simulink subsystem "BatteryTableBased"  (R2024b)
settings: Solver=VariableStepAuto  StartTime=0.0  StopTime=10.0  RelTol=1e-3
undefined symbols (not defined in the file or in its folder): battery
libraries: fl_lib x17, nesl_utility x9, batteryecm_lib x1, simulink x1
Description:
  | Battery Table-Based (Thermal)
  | 
  | ⚡ Main Features:
  | - Positive & negative relays for HV bus connection
  | - Electrical behavior from lookup tables (SOC–OCV, resistance vs SOC/Temp)
  | - Thermal port for coolant/heater coupling
  | - Voltage & current sensors for measurement
  | - Status bus bundles key signals
  | 
  | 📤 Outputs: Voltage, Current, SOC, Cell Voltage, Temperature
  | 
  | 📌 Use Case: High-fidelity drive cycle and thermal management studies
settings Model: Creator=isaacito  LastModifiedBy=jjha
settings OptimizationCC: ReuseModelBlockBuffer=off
settings RTWCC: GPUComputeCapability=3.5

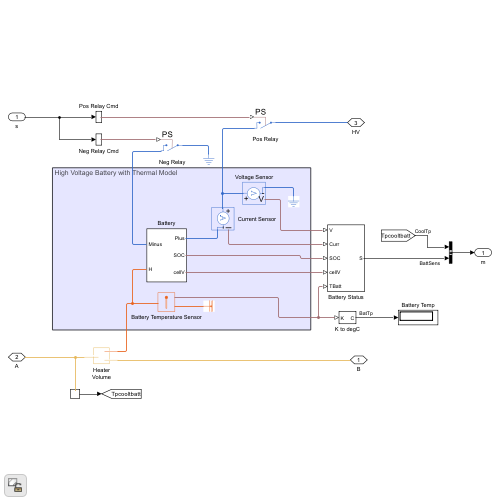
[thumbnail: Simulink's stored preview of the top-level diagram]
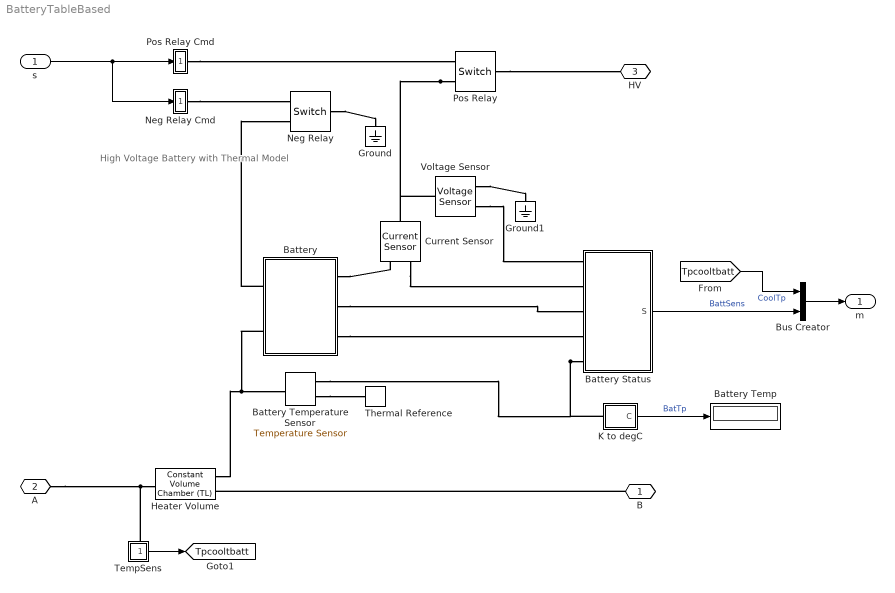
== system BatteryTableBased ==
  note: High Voltage Battery with Thermal Model
  s : Inport
  Battery : Subsystem
  Battery Status : Subsystem
  Battery Temp : Display
  Battery Temperature Sensor : fl_lib/Thermal/Thermal Sensors/Temperature Sensor  temperature_measure=foundation.enum.MeasurementReference.difference
  Bus Creator : BusCreator  Inputs=2
  Current Sensor : fl_lib/Electrical/Electrical Sensors/Current Sensor
  Ground : fl_lib/Electrical/Electrical Elements/Electrical Reference
  Ground1 : fl_lib/Electrical/Electrical Elements/Electrical Reference
  Heater Volume : fl_lib/Thermal Liquid/Elements/Constant Volume Chamber (TL)  volume=0.003 m^3  num_ports=foundation.enum.num_ports.two  area_A=pi * battery.coolant_pipe_D^2 / 4 m^2  area_B=pi * battery.coolant_pipe_D^2 / 4 m^2  area_C=0.01 m^2  area_D=0.01 m^2  p_I_specify=on  p_I_priority=High  p_I=vehicleThermal.coolant_p_init MPa  p_I_nominal_specify=off  p_I_nominal_value=1  p_I_nominal_unit=MPa  T_I_specify=on  T_I_priority=Low  T_I=vehicleThermal.coolant_T_init K  T_I_nominal_specify=off  T_I_nominal_value=1  T_I_nominal_unit=K  u_I_specify=off  u_I_priority=None  u_I=83.90600000000001 kJ/kg  u_I_nominal_specify=off  u_I_nominal_value=1  u_I_nominal_unit=kJ/kg  rho_I_specify=off  rho_I_priority=None  rho_I=998.21 kg/m^3  rho_I_nominal_specify=off  rho_I_nominal_value=1  rho_I_nominal_unit=kg/m^3
      settings: InternalSimscapePortConfiguration="{\"Bottom\":[],\"Left\":[{\"id\":\"A\",\"label\":\"A\",\"type\":\"foundation.thermal_liquid.thermal_liquid\"},{\"id\":\"H\",\"label\":\"H\",\"type\":\"foundation.thermal.thermal\"}],\"Right\":[{\"id\":\"B\",\"label\":\"B\",\"type\":\"foundation.thermal_liquid.thermal_liquid\"}],\"Top\":[]}"
  K to degC : Subsystem
  Neg Relay : fl_lib/Electrical/Electrical Elements/Switch  R_closed=0.001 Ohm  G_open=1e-8 1/Ohm  Threshold=0.5  i_specify=off  i_priority=None  i=0 A  i_nominal_specify=off  i_nominal_value=1  i_nominal_unit=A  v_specify=off  v_priority=None  v=0 V  v_nominal_specify=off  v_nominal_value=1  v_nominal_unit=V
  Neg Relay Cmd : Subsystem
  Pos Relay : fl_lib/Electrical/Electrical Elements/Switch  R_closed=0.001 Ohm  G_open=1e-8 1/Ohm  Threshold=0.5  i_specify=off  i_priority=None  i=0 A  i_nominal_specify=off  i_nominal_value=1  i_nominal_unit=A  v_specify=off  v_priority=None  v=0 V  v_nominal_specify=off  v_nominal_value=1  v_nominal_unit=V
  Pos Relay Cmd : Subsystem
  TempSens : Subsystem
      settings: PortSchema="{\"entries\":[{\"content\":{\"sides\":[{\"content\":{\"connectorIds\":[]},\"type\":\"ConnectorPlacement.EquallySpacedRectSide\",\"uuid\":\"72721b76-a3c2-4898-b03f-ac2748712f42\"},{\"content\":{\"connectorIds\":[\"Out1\"],\"side\":\"RIGHT\"},\"type\":\"ConnectorPlacement.EquallySpacedRectSide\",\"uuid\":\"bc8f9114-f4be-4e78-a030-a27ecd6c9d73\"},{\"content\":{\"connectorIds\":[\"LConn1\"],\"side\":\"TOP\"},\"type\":\"ConnectorPlacement.EquallySpacedRectSide\",\"uuid\":\"2039c7b0-1e2d-4162-8de8-f9f63ba2bad7\"}]},\"type\":\"ConnectorPlacement.EquallySpacedConnector\",\"uuid\":\"7ff72b7c-043d-4221-97f0-b3933d031f4d\"}],\"packageUris\":[\"http://schema.mathworks.com/mf0/Connector/R2020b\"],\"version\":\"1.0\"}"
  Thermal Reference : fl_lib/Thermal/Thermal Elements/Thermal Reference
  Voltage Sensor : fl_lib/Electrical/Electrical Sensors/Voltage Sensor
  B : PMIOPort  Side=Left
  A : PMIOPort  Port=2  Side=Right
  HV : PMIOPort  Port=3  Side=Right
  m : Outport
  tag scope: Tpcooltbatt=global
  wires:
  s/1 -> Neg Relay Cmd/1("  "), Pos Relay Cmd/1("  ")
  TempSens/1("  ") -> [Tpcooltbatt]
  [Tpcooltbatt] -> Bus Creator/1  "CoolTp"
  Bus Creator/1 -> m/1
  Battery Status/1(S) -> Bus Creator/2  "BattSens"
  K to degC/1(C) -> Battery Temp/1  "BatTp"
  connections:
  Pos Relay/RConn2 -- Current Sensor/LConn1 -- Voltage Sensor/LConn1
  Heater Volume/LConn2 -- Battery Temperature Sensor/LConn1 -- Battery/RConn2
  Battery Status/LConn5 -- K to degC/LConn1 -- Battery Temperature Sensor/RConn2
  TempSens/LConn1 -- A/RConn1 -- Heater Volume/RConn1
  Battery/RConn1 -- Neg Relay/RConn2
  Voltage Sensor/RConn1 -- Battery Status/LConn1
  Battery Temperature Sensor/RConn1 -- Thermal Reference/LConn1
  Battery/LConn2 -- Battery Status/LConn3
  Pos Relay Cmd/RConn1 -- Pos Relay/RConn1
  Neg Relay Cmd/RConn1 -- Neg Relay/RConn1
  Neg Relay/LConn1 -- Ground/LConn1
  B/RConn1 -- Heater Volume/LConn1
  Battery/LConn3 -- Battery Status/LConn4
  Pos Relay/LConn1 -- HV/RConn1
  Battery/LConn1 -- Current Sensor/RConn2
  Current Sensor/RConn1 -- Battery Status/LConn2
  Voltage Sensor/RConn2 -- Ground1/LConn1

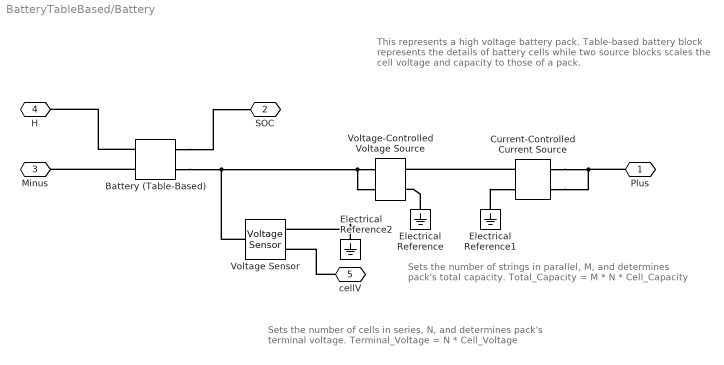
== system BatteryTableBased/Battery ==
  note: This represents a high voltage battery pack.
      | Table-based battery block represents the details of
      | battery cells while two source blocks scales
      | the cell voltage and capacity to those of a pack.
  note: Sets the number of strings in parallel, M,
      | and determines pack's total capacity.
      | Total_Capacity = M * N * Cell_Capacity
  note: Sets the number of cells in series, N,
      | and determines pack's terminal voltage.
      | Terminal_Voltage = N * Cell_Voltage
  Battery (Table-Based) : batteryecm_lib/Battery (Table-Based)  SOC_vec=battery.SOC_vec  T_dependence=simscape.enum.tablebattery.temperature_dependence.yes  prm_dir=simscape.enum.tablebattery.prm_dir.noCurrentDirectionality  T_vec=battery.T_vec K  V0_mat=battery.V0_mat V  V0_vec=[3.5057, 3.566, 3.6337, 3.7127, 3.9259, 4.0777, 4.1928] V  V_range=[0, inf] V  R0_mat=battery.R0_mat Ohm  R0_vec=[.0085, .0085, .0087, .0082, .0083, .0085, .0085] Ohm  R0_dis_mat=[.0117, .0085, .009; .011, .0085, .009; .0114, .0087, .0092; .0107, .0082, .0088; .0107, .0083, .0091; .0113, .0085, .0089; .0116, .0085, .0089] Ohm  R0_dis_vec=[.0085, .0085, .0087, .0082, .0083, .0085, .0085] Ohm  R0_ch_mat=[.0117, .0085, .009; .011, .0085, .009; .0114, .0087, .0092; .0107, .0082, .0088; .0107, .0083, .0091; .0113, .0085, .0089; .0116, .0085, .0089] Ohm  R0_ch_vec=[.0085, .0085, .0087, .0082, .0083, .0085, .0085] Ohm  AH=battery.AH A*hr  prm_leak=simscape.enum.tablebattery.prm_leak.disabled  Rleak_vec=[8000, 7000, 6000] Ohm  Rleak=7e3 Ohm  extrapolation_option=simscape.enum.extrapolation.nearest  SOC_port=simscape.enum.tablebattery.enable.yes  prm_dyn=simscape.enum.tablebattery.prm_dyn.off  R1_mat=[.0109, .0029, .0013; .0069, .0024, .0012; .0047, .0026, .0013; .0034, .0016, .001; .0033, .0023, .0014; .0033, .0018, .0011; .0028, .0017, .0011] Ohm  R1_vec=[.0029, .0024, .0026, .0016, .0023, .0018, .0017] Ohm  tau1_mat=[20, 36, 39; 31, 45, 39; 109, 105, 61; 36, 29, 26; 59, 77, 67; 40, 33, 29; 25, 39, 33] s  tau1_vec=[36, 45, 105, 29, 77, 33, 39] s  R2_mat=[.0109, .0029, .0013; .0069, .0024, .0012; .0047, .0026, .0013; .0034, .0016, .001; .0033, .0023, .0014; .0033, .0018, .0011; .0028, .0017, .0011] Ohm  R2_vec=[.0029, .0024, .0026, .0016, .0023, .0018, .0017] Ohm  tau2_mat=[20, 36, 39; 31, 45, 39; 109, 105, 61; 36, 29, 26; 59, 77, 67; 40, 33, 29; 25, 39, 33] s  tau2_vec=[36, 45, 105, 29, 77, 33, 39] s  R3_mat=[.0109, .0029, .0013; .0069, .0024, .0012; .0047, .0026, .0013; .0034, .0016, .001; .0033, .0023, .0014; .0033, .0018, .0011; .0028, .0017, .0011] Ohm  R3_vec=[.0029, .0024, .0026, .0016, .0023, .0018, .0017] Ohm  tau3_mat=[20, 36, 39; 31, 45, 39; 109, 105, 61; 36, 29, 26; 59, 77, 67; 40, 33, 29; 25, 39, 33] s  tau3_vec=[36, 45, 105, 29, 77, 33, 39] s  R4_mat=[.0109, .0029, .0013; .0069, .0024, .0012; .0047, .0026, .0013; .0034, .0016, .001; .0033, .0023, .0014; .0033, .0018, .0011; .0028, .0017, .0011] Ohm  R4_vec=[.0029, .0024, .0026, .0016, .0023, .0018, .0017] Ohm  tau4_mat=[20, 36, 39; 31, 45, 39; 109, 105, 61; 36, 29, 26; 59, 77, 67; 40, 33, 29; 25, 39, 33] s  tau4_vec=[36, 45, 105, 29, 77, 33, 39] s  R5_mat=[.0109, .0029, .0013; .0069, .0024, .0012; .0047, .0026, .0013; .0034, .0016, .001; .0033, .0023, .0014; .0033, .0018, .0011; .0028, .0017, .0011] Ohm  R5_vec=[.0029, .0024, .0026, .0016, .0023, .0018, .0017] Ohm  tau5_mat=[20, 36, 39; 31, 45, 39; 109, 105, 61; 36, 29, 26; 59, 77, 67; 40, 33, 29; 25, 39, 33] s  tau5_vec=[36, 45, 105, 29, 77, 33, 39] s  prm_fade=simscape.enum.tablebattery.prm_fade.disabled  N0=100  dV0=0  dR0=0  dAH=0  dRleak=0  dR1=0  dR2=0  dR3=0  dR4=0  dR5=0  N0vec=[100, 200, 300]  Tfadevec=[298.15, 323.15] K  dV0vec=[0, 0, 0]  dR0vec=[0, 0, 0]  dAHvec=[0, 0, 0]  dRleakvec=[0, 0, 0]  dR1vec=[0, 0, 0]  dR2vec=[0, 0, 0]  dR3vec=[0, 0, 0]  dR4vec=[0, 0, 0]  dR5vec=[0, 0, 0]  dV0mat=[0, 0; 0, 0; 0, 0]  dR0mat=[0, 0; 0, 0; 0, 0]  dAHmat=[0, 0; 0, 0; 0, 0]  dRleakmat=[0, 0; 0, 0; 0, 0]  dR1mat=[0, 0; 0, 0; 0, 0]  dR2mat=[0, 0; 0, 0; 0, 0]  dR3mat=[0, 0; 0, 0; 0, 0]  dR4mat=[0, 0; 0, 0; 0, 0]  dR5mat=[0, 0; 0, 0; 0, 0]  prm_age_modeling=simscape.enum.tablebattery.prm_age_modeling.equation  storage_dt_age_vec=[0] d  storage_T_age_vec=[273] K  prm_age_OCV=simscape.enum.tablebattery.prm_age_OCV.OCV  OCV_age=0.9  SOC_age=0.6  prm_age_resistance=simscape.enum.tablebattery.prm_age.disabled  OCV_scaling_age_resistance=2.2134e6  OCV_offset_age_resistance=1.632e6  temp_exp_age_resistance=0.515833569 V  t_exp_age_resistance=0.75  T_age_vec_resistance=[273.15, 298.15, 323.15] K  dt_age_vec_resistance=[90, 180, 270, 360] d  dR0_age_vec=[0, 0, 0]  t_meas_dR0_age=100 d  dR0_age_mat=[0, 0, 0; 0, 0, 0; 0, 0, 0; 0, 0, 0]  prm_age_capacity=simscape.enum.tablebattery.prm_age.disabled  OCV_scaling_age_capacity=1.5097e07  OCV_offset_age_capacity=8.3625e06  temp_exp_age_capacity=0.6011 V  t_exp_age_capacity=0.75  T_age_vec_capacity=[273.15, 298.15, 323.15] K  dt_age_vec_capacity=[90, 180, 270, 360] d  dAH_age_vec=[0, 0, 0]  t_meas_dAH_age=100 d  dAH_age_mat=[0, 0, 0; 0, 0, 0; 0, 0, 0; 0, 0, 0]  thermal_port=simscape.enum.thermaleffects.model  temperature=298.15 K  thermal_mass=battery.Ns J/K  i_specify=off  i_priority=None  i=0 A  i_nominal_specify=off  i_nominal_value=1  i_nominal_unit=A  v_specify=off  v_priority=None  v=0 V  v_nominal_specify=off  v_nominal_value=1  v_nominal_unit=V  stateOfCharge_specify=on  stateOfCharge_priority=High  stateOfCharge=battery.initialPackSOC  stateOfCharge_nominal_specify=off  stateOfCharge_nominal_value=1  stateOfCharge_nominal_unit=1  num_cycles_specify=off  num_cycles_priority=High  num_cycles=0  num_cycles_nominal_specify=off  num_cycles_nominal_value=1  num_cycles_nominal_unit=1  cell_temperature_specify=on  cell_temperature_priority=Low  cell_temperature=vehicleThermal.ambient K  cell_temperature_nominal_specify=off  cell_temperature_nominal_value=1  cell_temperature_nominal_unit=K
  Current-Controlled Current Source : fl_lib/Electrical/Electrical Sources/Current-Controlled Current Source  K=battery.Np*-1  i1_specify=off  i1_priority=None  i1=0 A  i1_nominal_specify=off  i1_nominal_value=1  i1_nominal_unit=A  i2_specify=off  i2_priority=None  i2=0 A  i2_nominal_specify=off  i2_nominal_value=1  i2_nominal_unit=A
      settings: InternalSimscapePortConfiguration="{\"Bottom\":[],\"Left\":[{\"id\":\"p1\",\"label\":\"+\",\"type\":\"foundation.electrical.electrical\"},{\"id\":\"head\",\"label\":\"\",\"type\":\"foundation.electrical.electrical\"}],\"Right\":[{\"id\":\"n1\",\"label\":\"-\",\"type\":\"foundation.electrical.electrical\"},{\"id\":\"tail\",\"label\":\"\",\"type\":\"foundation.electrical.electrical\"}],\"Top\":[]}"
  Electrical Reference : fl_lib/Electrical/Electrical Elements/Electrical Reference
  Electrical Reference1 : fl_lib/Electrical/Electrical Elements/Electrical Reference
  Electrical Reference2 : fl_lib/Electrical/Electrical Elements/Electrical Reference
  Voltage Sensor : fl_lib/Electrical/Electrical Sensors/Voltage Sensor
  Voltage-Controlled Voltage Source : fl_lib/Electrical/Electrical Sources/Voltage-Controlled Voltage Source  K=battery.Ns*-1  v1_specify=off  v1_priority=None  v1=0 V  v1_nominal_specify=off  v1_nominal_value=1  v1_nominal_unit=V  v2_specify=off  v2_priority=None  v2=0 V  v2_nominal_specify=off  v2_nominal_value=1  v2_nominal_unit=V
      settings: InternalSimscapePortConfiguration="{\"Bottom\":[],\"Left\":[{\"id\":\"p1\",\"label\":\"+\",\"type\":\"foundation.electrical.electrical\"},{\"id\":\"p2\",\"label\":\"+\",\"type\":\"foundation.electrical.electrical\"}],\"Right\":[{\"id\":\"n1\",\"label\":\"-\",\"type\":\"foundation.electrical.electrical\"},{\"id\":\"n2\",\"label\":\"-\",\"type\":\"foundation.electrical.electrical\"}],\"Top\":[]}"
  Plus : PMIOPort  Side=Left
  SOC : PMIOPort  Port=2  Side=Left
  Minus : PMIOPort  Port=3  Side=Right
  H : PMIOPort  Port=4  Side=Right
  cellV : PMIOPort  Port=5  Side=Left
  connections:
  Electrical Reference1/LConn1 -- Current-Controlled Current Source/LConn2
  Electrical Reference/LConn1 -- Voltage-Controlled Voltage Source/LConn1
  Voltage Sensor/LConn1 -- Battery (Table-Based)/LConn1 -- Voltage-Controlled Voltage Source/RConn1 -- Voltage-Controlled Voltage Source/RConn2
  Current-Controlled Current Source/LConn1 -- Voltage-Controlled Voltage Source/LConn2
  Plus/RConn1 -- Current-Controlled Current Source/RConn1 -- Current-Controlled Current Source/RConn2
  Battery (Table-Based)/RConn1 -- Minus/RConn1
  Battery (Table-Based)/LConn2 -- SOC/RConn1
  Battery (Table-Based)/RConn2 -- H/RConn1
  Electrical Reference2/LConn1 -- Voltage Sensor/RConn2
  cellV/RConn1 -- Voltage Sensor/RConn1

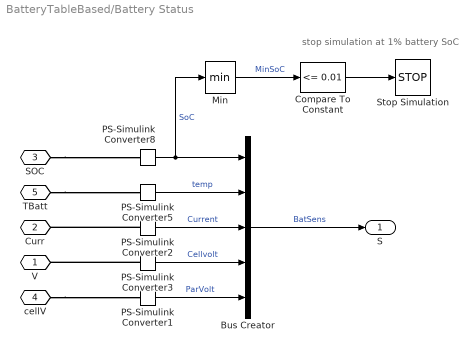
== system BatteryTableBased/Battery Status ==
  note: stop simulation at 1% battery SoC
  Bus Creator : BusCreator  Inputs=5
  Compare To Constant : simulink/Logic and Bit Operations/Compare To Constant  relop=<=  const=0.01  OutDataTypeStr=boolean
  Min : MinMax
  PS-Simulink Converter1 : nesl_utility/PS-Simulink Converter  PhysicalDomain=network_engine_domain  SubClassName=ps_output  LeftPortType=input  RightPortType=output  PseudoPeriodic=off  Frequencies=[]  VectorFormat=1-D array  Unit=V  AffineConversion=off
  PS-Simulink Converter2 : nesl_utility/PS-Simulink Converter  PhysicalDomain=network_engine_domain  SubClassName=ps_output  LeftPortType=input  RightPortType=output  PseudoPeriodic=off  Frequencies=[]  VectorFormat=1-D array  Unit=A  AffineConversion=off
  PS-Simulink Converter3 : nesl_utility/PS-Simulink Converter  PhysicalDomain=network_engine_domain  SubClassName=ps_output  LeftPortType=input  RightPortType=output  PseudoPeriodic=off  Frequencies=[]  VectorFormat=1-D array  Unit=V  AffineConversion=off
  PS-Simulink Converter5 : nesl_utility/PS-Simulink Converter  PhysicalDomain=network_engine_domain  SubClassName=ps_output  LeftPortType=input  RightPortType=output  PseudoPeriodic=off  Frequencies=[]  VectorFormat=inherit  Unit=K  AffineConversion=on
  PS-Simulink Converter8 : nesl_utility/PS-Simulink Converter  PhysicalDomain=network_engine_domain  SubClassName=ps_output  LeftPortType=input  RightPortType=output  PseudoPeriodic=off  Frequencies=[]  VectorFormat=1-D array  Unit=1  AffineConversion=off
  Stop Simulation : Stop
  V : PMIOPort  Side=Left
  Curr : PMIOPort  Port=2  Side=Left
  SOC : PMIOPort  Port=3  Side=Left
  cellV : PMIOPort  Port=4  Side=Left
  TBatt : PMIOPort  Port=5  Side=Left
  S : Outport
  wires:
  PS-Simulink Converter5/1 -> Bus Creator/2  "temp"
  PS-Simulink Converter2/1 -> Bus Creator/3  "Current"
  PS-Simulink Converter3/1 -> Bus Creator/4  "Cellvolt"
  Compare To Constant/1 -> Stop Simulation/1
  Min/1 -> Compare To Constant/1  "MinSoC"
  PS-Simulink Converter8/1 -> Min/1, Bus Creator/1  "SoC"
  PS-Simulink Converter1/1 -> Bus Creator/5  "ParVolt"
  Bus Creator/1 -> S/1  "BatSens"
  connections:
  TBatt/RConn1 -- PS-Simulink Converter5/LConn1
  SOC/RConn1 -- PS-Simulink Converter8/LConn1
  PS-Simulink Converter2/LConn1 -- Curr/RConn1
  PS-Simulink Converter3/LConn1 -- V/RConn1
  cellV/RConn1 -- PS-Simulink Converter1/LConn1

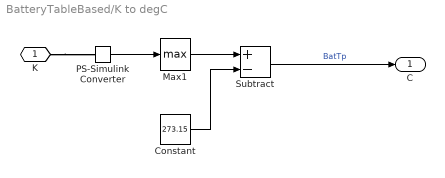
== system BatteryTableBased/K to degC ==
  Constant : Constant  Value=273.15
  Max1 : MinMax  Function=max
  PS-Simulink Converter : nesl_utility/PS-Simulink Converter  PhysicalDomain=network_engine_domain  SubClassName=ps_output  LeftPortType=input  RightPortType=output  PseudoPeriodic=off  Frequencies=[]  VectorFormat=inherit  Unit=K  AffineConversion=off
  Subtract : Sum  Inputs=+-
  K : PMIOPort  Side=Left
  C : Outport
  wires:
  PS-Simulink Converter/1 -> Max1/1
  Max1/1 -> Subtract/1
  Subtract/1 -> C/1  "BatTp"
  Constant/1 -> Subtract/2
  connections:
  K/RConn1 -- PS-Simulink Converter/LConn1

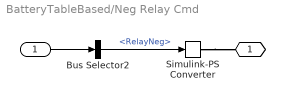
== system BatteryTableBased/Neg Relay Cmd ==
  "  " : Inport
  Bus Selector2 : BusSelector  OutputSignals=RelayNeg
  Simulink-PS Converter : nesl_utility/Simulink-PS Converter  PhysicalDomain=network_engine_domain  SubClassName=ps_input  LeftPortType=input  RightPortType=output  PseudoPeriodic=off  Frequencies=[]  NoiseDistribution=none  NoiseParameters=[]  Unit=1  AffineConversion=off  FilteringAndDerivatives=provide  SimscapeFilterOrder=1  InputFilterTimeConstant=0.001  UdotUserProvided=0
  " " : PMIOPort  Side=Right
  wires:
  "  "/1 -> Bus Selector2/1
  Bus Selector2/1 -> Simulink-PS Converter/1  "<RelayNeg>"
  connections:
  Simulink-PS Converter/RConn1 -- " "/RConn1

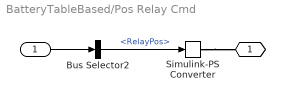
== system BatteryTableBased/Pos Relay Cmd ==
  "  " : Inport
  Bus Selector2 : BusSelector  OutputSignals=RelayPos
  Simulink-PS Converter : nesl_utility/Simulink-PS Converter  PhysicalDomain=network_engine_domain  SubClassName=ps_input  LeftPortType=input  RightPortType=output  PseudoPeriodic=off  Frequencies=[]  NoiseDistribution=none  NoiseParameters=[]  Unit=1  AffineConversion=off  FilteringAndDerivatives=provide  SimscapeFilterOrder=1  InputFilterTimeConstant=0.001  UdotUserProvided=0
  " " : PMIOPort  Side=Right
  wires:
  Bus Selector2/1 -> Simulink-PS Converter/1  "<RelayPos>"
  "  "/1 -> Bus Selector2/1
  connections:
  Simulink-PS Converter/RConn1 -- " "/RConn1

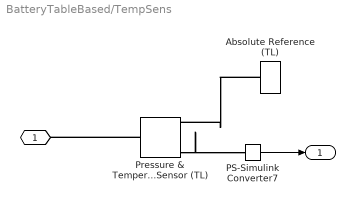
== system BatteryTableBased/TempSens ==
  Absolute Reference (TL) : fl_lib/Thermal Liquid/Elements/Absolute Reference (TL)
  PS-Simulink Converter7 : nesl_utility/PS-Simulink Converter  PhysicalDomain=network_engine_domain  SubClassName=ps_output  LeftPortType=input  RightPortType=output  PseudoPeriodic=off  Frequencies=[]  VectorFormat=inherit  Unit=inherit  AffineConversion=off
  Pressure & Temperature Sensor (TL) : fl_lib/Thermal Liquid/Sensors/Pressure & Temperature Sensor (TL)  reference=foundation.enum.MeasurementReference.difference  pressure=true  pressure_spec=foundation.enum.PressureMeasementSpec.Absolute  temperature=true
      settings: InternalSimscapePortConfiguration="{\"Bottom\":[{\"id\":\"T\",\"label\":\"T\",\"type\":\"output\"}],\"Left\":[{\"id\":\"A\",\"label\":\"A\",\"type\":\"foundation.thermal_liquid.thermal_liquid\"}],\"Right\":[{\"id\":\"B\",\"label\":\"B\",\"type\":\"foundation.thermal_liquid.thermal_liquid\"},{\"id\":\"P\",\"label\":\"P\",\"type\":\"output\"}],\"Top\":[]}"
  " " : PMIOPort  Side=Left
  "  " : Outport
  wires:
  PS-Simulink Converter7/1 -> "  "/1
  connections:
  Pressure & Temperature Sensor (TL)/RConn3 -- PS-Simulink Converter7/LConn1
  Absolute Reference (TL)/LConn1 -- Pressure & Temperature Sensor (TL)/RConn1
  Pressure & Temperature Sensor (TL)/LConn1 -- " "/RConn1
